simulink model "sampleModel2002_1_sub_sub"  (R2023a)
settings: Solver=VariableStepAuto  StartTime=0.0  StopTime=10.0  RelTol=1e-3
libraries: hdlsllib x9
settings Model: Creator=user1  LastModifiedBy=user1

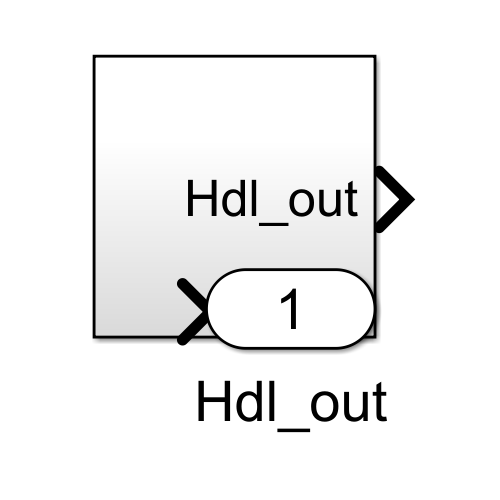
[thumbnail: Simulink's stored preview of the top-level diagram]
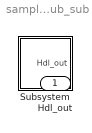
== system sampleModel2002_1_sub_sub ==
  Subsystem : Subsystem
  Hdl_out : Outport  OutDataTypeStr=uint8

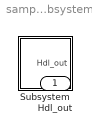
== system sampleModel2002_1_sub_sub/Subsystem ==
  Subsystem : Subsystem
  Hdl_out : Outport  OutDataTypeStr=uint8

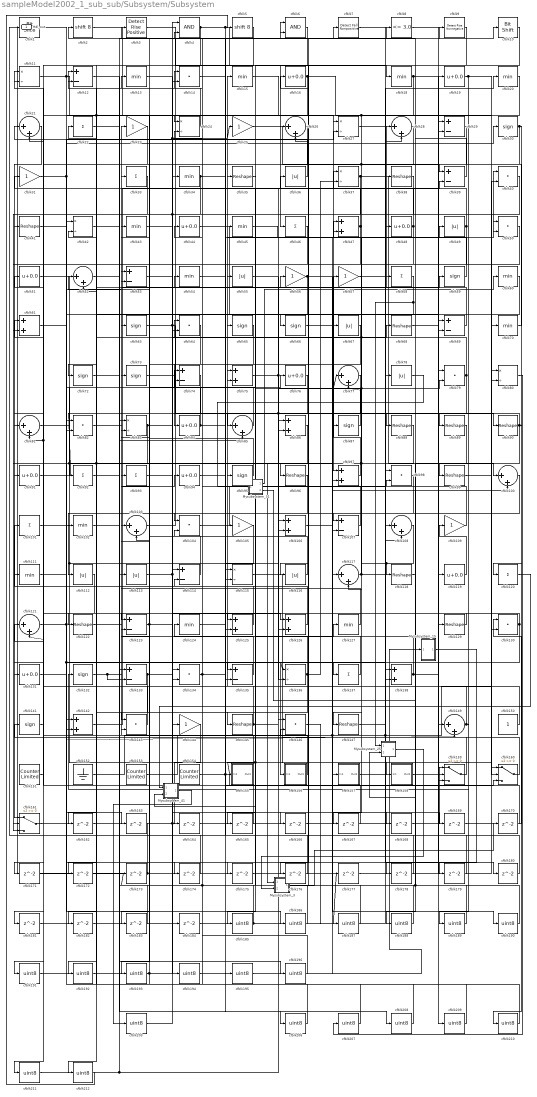
== system sampleModel2002_1_sub_sub/Subsystem/Subsystem ==
  Mysubsystem_15 : Subsystem  TreatAsAtomicUnit=on  RTWFcnName=Mysubsystem_15
      settings: RTWFcnNameOpts=User specified  RTWFileNameOpts=Use function name
  Mysubsystem_25 : Subsystem  TreatAsAtomicUnit=on  RTWFcnName=Mysubsystem_25
      settings: RTWFcnNameOpts=User specified  RTWFileNameOpts=Use function name
  Mysubsystem_3 : Subsystem  TreatAsAtomicUnit=on  RTWFcnName=Mysubsystem_3
      settings: RTWFcnNameOpts=User specified  RTWFileNameOpts=Use function name
  Mysubsystem_31 : Subsystem  TreatAsAtomicUnit=on  RTWFcnName=Mysubsystem_31
      settings: RTWFcnNameOpts=User specified  RTWFileNameOpts=Use function name
  Mysubsystem_41 : Subsystem  TreatAsAtomicUnit=on  RTWFcnName=Mysubsystem_41
      settings: RTWFcnNameOpts=User specified  RTWFileNameOpts=Use function name
  cfblk1 : hdlsllib/Logic and Bit Operations/Bit Slice  lidx=7  ridx=0
  cfblk10 : hdlsllib/Logic and Bit Operations/Bit Shift  mode=Shift Left Logical  N=0
  cfblk{21,26,28,52,77,81,85,100,103,108,117,121,149} (13 alike) : Sum  Inputs=|++  OutDataTypeStr=uint8
  cfblk{22,33,46,58,92..93,101,120,137} (9 alike) : Sum  Inputs=+  OutDataTypeStr=uint8
  cfblk{13,15,18,20,34,43,45,54,60,70,102,111,124,127} (14 alike) : MinMax  OutDataTypeStr=uint8
  cfblk{14,40,50,64,79,82,98,104,130,134,143,146} (12 alike) : DotProduct  OutDataTypeStr=uint8
  cfblk{23,25,31,56..57,105,109,144} (8 alike) : Gain  OutDataTypeStr=uint8
  cfblk{47,61,75,86,97,106,125..126,138,142} (10 alike) : Sum  OutDataTypeStr=uint8
  cfblk{12,29,39,53,69,74,107,114,123,133,135} (11 alike) : Sum  Inputs=+-  OutDataTypeStr=uint8
  cfblk{11,24,27,37,42,80,83,115,136} (9 alike) : Product  Inputs=*/  OutDataTypeStr=uint8  RndMeth=Zero  SaturateOnIntegerOverflow=on
  cfblk{36,49,55,67,78,112..113,116} (8 alike) : Abs  OutDataTypeStr=uint8  SaturateOnIntegerOverflow=off
  cfblk{35,38,41,68,88..90,96,99,118,122,129,145,147} (14 alike) : Reshape
  cfblk{16,19,44,48,51,76,84,91,94,119,131} (11 alike) : Bias  Bias=0.0  SaturateOnIntegerOverflow=off
  cfblk{30,59,63,65..66,72..73,87,95,132,141} (11 alike) : Signum
  cfblk150 : Constant  OutDataTypeStr=uint8  SampleTime=-1
  cfblk151 : hdlsllib/Sources/Counter Limited  uplimit=7  tsamp=-1
  cfblk152 : Ground
  cfblk153 : hdlsllib/Sources/Counter Limited  uplimit=7  tsamp=-1
  cfblk154 : hdlsllib/Sources/Counter Limited  uplimit=7  tsamp=-1
  cfblk155 : Subsystem
      settings: LibrarySourceBlock=|
      | hdlsllib/Ports &
      | Subsystems/Subsystem
  cfblk156 : Subsystem
      settings: LibrarySourceBlock=|
      | hdlsllib/Ports &
      | Subsystems/Subsystem
  cfblk157 : Subsystem
      settings: LibrarySourceBlock=|
      | hdlsllib/Ports &
      | Subsystems/Subsystem
  cfblk158 : Subsystem
      settings: LibrarySourceBlock=|
      | hdlsllib/Ports &
      | Subsystems/Subsystem
  cfblk159 : Switch  OutDataTypeStr=uint8  SaturateOnIntegerOverflow=off  InputSameDT=off
  cfblk160 : Switch  OutDataTypeStr=uint8  SaturateOnIntegerOverflow=off  InputSameDT=off
  cfblk161 : Switch  OutDataTypeStr=uint8  SaturateOnIntegerOverflow=off  InputSameDT=off
  cfblk{162..184} (23 alike) : Delay  SampleTime=1
  cfblk{185..196,203,206..212} (20 alike) : DataTypeConversion  OutDataTypeStr=uint8  SaturateOnIntegerOverflow=off  RndMeth=Floor
  cfblk2 : ArithShift  BitShiftNumber=8
  cfblk3 : hdlsllib/Logic and Bit Operations/Detect Rise Positive  vinit=0  OutDataTypeStr=uint8
  cfblk4 : Logic  AllPortsSameDT=off  OutDataTypeStr=boolean
  cfblk5 : ArithShift  BitShiftNumber=8
  cfblk6 : Logic  AllPortsSameDT=off  OutDataTypeStr=boolean
  cfblk7 : hdlsllib/Logic and Bit Operations/Detect Fall Nonpositive  vinit=0  OutDataTypeStr=uint8
  cfblk8 : hdlsllib/Logic and Bit Operations/Compare To Constant  relop=<=  const=3.0  OutDataTypeStr=uint8
  cfblk9 : hdlsllib/Logic and Bit Operations/Detect Rise Nonnegative  vinit=0  OutDataTypeStr=uint8
  Hdl_out : Outport  OutDataTypeStr=uint8
  wires:
  Mysubsystem_41/1(Out1) -> cfblk203/1
  cfblk120/1 -> Mysubsystem_41/1(In1)
  Mysubsystem_31/2(Out2) -> Mysubsystem_25/2(In2)
  Mysubsystem_31/1(Out1) -> cfblk60/1
  cfblk78/1 -> Mysubsystem_31/1(In1)
  Mysubsystem_25/1(Out1) -> Mysubsystem_3/2(In2)
  Mysubsystem_15/1(Out1) -> cfblk178/1
  cfblk195/1 -> Mysubsystem_15/1(In1)
  Mysubsystem_3/1(Out1) -> cfblk170/1
  cfblk212/1 -> cfblk5/1
  cfblk211/1 -> cfblk86/2, cfblk113/1
  cfblk210/1 -> cfblk42/2
  cfblk209/1 -> cfblk42/1
  cfblk8/1 -> cfblk209/1
  cfblk208/1 -> cfblk82/1
  cfblk42/1 -> cfblk208/1
  cfblk207/1 -> cfblk54/1
  cfblk80/1 -> cfblk207/1
  cfblk206/1 -> cfblk63/1
  cfblk54/1 -> cfblk206/1
  cfblk203/1 -> cfblk184/1
  cfblk196/1 -> cfblk124/1
  cfblk102/1 -> cfblk196/1
  cfblk124/1 -> cfblk195/1
  cfblk194/1 -> cfblk67/1
  cfblk43/1 -> cfblk194/1
  cfblk193/1 -> cfblk14/2, cfblk93/1
  cfblk192/1 -> cfblk106/2
  cfblk172/1 -> cfblk192/1
  cfblk191/1 -> cfblk106/1
  cfblk23/1 -> cfblk191/1
  cfblk190/1 -> cfblk98/2, cfblk43/1
  cfblk189/1 -> cfblk146/2
  cfblk188/1 -> cfblk146/1
  cfblk89/1 -> cfblk188/1
  cfblk187/1 -> cfblk173/1, cfblk104/2
  cfblk186/1 -> cfblk35/1
  cfblk61/1 -> cfblk186/1
  cfblk185/1 -> cfblk177/1, cfblk143/2
  cfblk184/1 -> cfblk117/1
  cfblk183/1 -> cfblk83/1
  cfblk182/1 -> cfblk133/1
  cfblk181/1 -> cfblk138/1
  cfblk26/1 -> cfblk181/1
  cfblk180/1 -> cfblk115/1
  cfblk27/1 -> cfblk180/1
  cfblk179/1 -> cfblk74/2
  cfblk178/1 -> cfblk123/2
  cfblk177/1 -> cfblk149/1
  cfblk176/1 -> cfblk24/2
  cfblk175/1 -> cfblk79/1
  cfblk52/1 -> cfblk175/1
  cfblk174/1 -> cfblk12/2
  cfblk173/1 -> cfblk142/1, Hdl_out/1
  cfblk171/1 -> cfblk130/2
  cfblk112/1 -> cfblk171/1
  cfblk170/1 -> cfblk103/1
  cfblk169/1 -> cfblk40/2
  cfblk157/1(Out1) -> cfblk169/1
  cfblk168/1 -> cfblk159/3
  cfblk14/1 -> cfblk168/1
  cfblk167/1 -> cfblk21/2
  cfblk166/1 -> cfblk29/2
  cfblk13/1 -> cfblk166/1
  cfblk165/1 -> cfblk121/1
  cfblk6/1 -> cfblk165/1
  cfblk164/1 -> cfblk108/2
  cfblk144/1 -> cfblk164/1
  cfblk163/1 -> cfblk1/1
  cfblk162/1 -> cfblk69/1
  cfblk46/1 -> cfblk61/2
  cfblk96/1 -> Mysubsystem_41/2(In2), cfblk155/1(In1)
  cfblk151/1 -> cfblk61/1
  cfblk90/1 -> cfblk87/1, cfblk99/1, cfblk120/1
  cfblk31/1 -> cfblk30/1, cfblk174/1
  cfblk50/1 -> cfblk135/2
  cfblk92/1 -> cfblk9/1
  cfblk147/1 -> cfblk20/1
  cfblk11/1 -> cfblk105/1, cfblk26/1
  cfblk7/1 -> cfblk98/1
  cfblk94/1 -> cfblk6/1
  cfblk66/1 -> cfblk50/1
  cfblk40/1 -> cfblk41/1
  cfblk58/1 -> Mysubsystem_25/1(In1), cfblk96/1
  cfblk60/1 -> cfblk117/2
  cfblk38/1 -> cfblk134/2, cfblk82/2
  cfblk20/1 -> cfblk103/2, cfblk77/2
  cfblk131/1 -> cfblk53/2
  cfblk22/1 -> cfblk138/2
  cfblk150/1 -> cfblk64/1
  cfblk123/1 -> cfblk126/1, cfblk83/2
  cfblk41/1 -> cfblk149/2, cfblk136/1
  cfblk99/1 -> cfblk80/2
  cfblk28/1 -> cfblk81/1, cfblk167/1
  cfblk24/1 -> cfblk12/1
  cfblk47/1 -> cfblk4/2, cfblk176/1
  cfblk117/1 -> cfblk77/1, cfblk47/2, cfblk48/1
  cfblk104/1 -> cfblk28/2
  cfblk83/1 -> cfblk59/1, cfblk131/1
  cfblk87/1 -> cfblk55/1
  cfblk12/1 -> cfblk85/2
  cfblk108/1 -> cfblk147/1, cfblk118/1
  cfblk49/1 -> cfblk116/1, cfblk11/2
  cfblk133/1 -> cfblk25/1, cfblk7/1, cfblk212/1
  cfblk160/1 -> cfblk141/1
  cfblk156/1(Out1) -> cfblk111/1
  cfblk111/1 -> cfblk27/2
  cfblk105/1 -> cfblk125/2
  cfblk69/1 -> cfblk22/1
  cfblk74/1 -> cfblk123/1
  cfblk55/1 -> cfblk86/1
  cfblk125/1 -> cfblk101/1
  cfblk15/1 -> cfblk27/1
  cfblk34/1 -> cfblk72/1, cfblk137/1
  cfblk19/1 -> cfblk160/1, cfblk189/1
  cfblk134/1 -> cfblk114/2, cfblk37/1
  cfblk95/1 -> cfblk53/1
  cfblk135/1 -> cfblk44/1
  cfblk143/1 -> cfblk31/1
  cfblk59/1 -> cfblk45/1
  cfblk116/1 -> cfblk52/1
  cfblk85/1 -> cfblk3/1
  cfblk65/1 -> cfblk143/1
  cfblk75/1 -> cfblk39/2, cfblk79/2
  cfblk142/1 -> cfblk127/1
  cfblk113/1 -> cfblk134/1, cfblk68/1
  cfblk35/1 -> cfblk185/1
  cfblk29/1 -> cfblk115/2
  cfblk64/1 -> cfblk84/1
  cfblk130/1 -> cfblk122/1, cfblk142/2
  cfblk33/1 -> cfblk161/3
  cfblk136/1 -> cfblk75/2, cfblk37/2, cfblk183/1
  cfblk100/1 -> cfblk112/1
  cfblk101/1 -> cfblk156/1(In1), cfblk126/2
  cfblk73/1 -> cfblk90/1
  cfblk3/1 -> cfblk108/1
  cfblk137/1 -> cfblk75/1
  cfblk67/1 -> cfblk193/1
  cfblk146/1 -> cfblk187/1
  cfblk98/1 -> cfblk104/1
  cfblk84/1 -> cfblk49/1, cfblk33/1
  cfblk129/1 -> cfblk125/1
  cfblk141/1 -> cfblk51/1
  cfblk5/1 -> cfblk211/1
  cfblk68/1 -> cfblk19/1
  cfblk56/1 -> cfblk100/2, cfblk172/1
  cfblk1/1 -> cfblk69/2
  cfblk10/1 -> cfblk18/1
  cfblk152/1 -> cfblk78/1, cfblk50/2, cfblk107/2
  cfblk18/1 -> cfblk121/2, cfblk81/2, cfblk162/1, cfblk160/2
  cfblk118/1 -> cfblk8/1
  cfblk30/1 -> cfblk89/1, cfblk210/1
  cfblk48/1 -> cfblk91/1, cfblk6/2
  cfblk36/1 -> cfblk13/1
  cfblk72/1 -> cfblk135/1
  cfblk138/1 -> cfblk29/1, cfblk26/2
  cfblk93/1 -> cfblk34/1
  cfblk161/1 -> cfblk130/1, cfblk4/1
  cfblk153/1 -> cfblk80/1
  cfblk126/1 -> cfblk95/1
  cfblk9/1 -> cfblk66/1
  cfblk76/1 -> cfblk145/1
  cfblk114/1 -> cfblk21/1
  cfblk79/1 -> cfblk52/2, cfblk47/1, cfblk88/1
  cfblk51/1 -> cfblk114/1
  cfblk109/1 -> cfblk14/1
  cfblk77/1 -> cfblk92/1, cfblk136/2
  cfblk86/1 -> cfblk161/2, cfblk182/1
  cfblk97/1 -> cfblk57/1
  cfblk37/1 -> cfblk100/1, cfblk64/2
  cfblk158/1(Out1) -> cfblk119/1
  cfblk16/1 -> cfblk24/1, cfblk70/1
  cfblk57/1 -> cfblk28/1
  cfblk159/1 -> cfblk16/1
  cfblk39/1 -> cfblk2/1
  cfblk25/1 -> cfblk129/1
  cfblk106/1 -> cfblk190/1
  cfblk149/1 -> cfblk132/1, cfblk11/1
  cfblk155/1(Out1) -> cfblk73/1
  cfblk91/1 -> cfblk76/1
  cfblk70/1 -> cfblk39/1
  cfblk115/1 -> cfblk159/2
  cfblk63/1 -> cfblk85/1, cfblk38/1
  cfblk53/1 -> cfblk144/1
  cfblk154/1 -> cfblk159/1, cfblk160/3
  cfblk81/1 -> cfblk158/1(In1), cfblk157/1(In1)
  cfblk122/1 -> cfblk36/1
  cfblk88/1 -> Mysubsystem_3/1(In1), cfblk107/1
  cfblk121/1 -> cfblk74/1, cfblk163/1
  cfblk44/1 -> cfblk97/2
  cfblk107/1 -> cfblk65/1
  cfblk82/1 -> cfblk56/1
  cfblk2/1 -> cfblk97/1
  cfblk21/1 -> cfblk161/1
  cfblk45/1 -> cfblk40/1
  cfblk132/1 -> cfblk94/1, cfblk133/2
  cfblk4/1 -> cfblk46/1, cfblk179/1, cfblk102/1
  cfblk145/1 -> cfblk15/1, cfblk58/1
  cfblk127/1 -> cfblk23/1
  cfblk119/1 -> cfblk109/1
  cfblk103/1 -> cfblk10/1

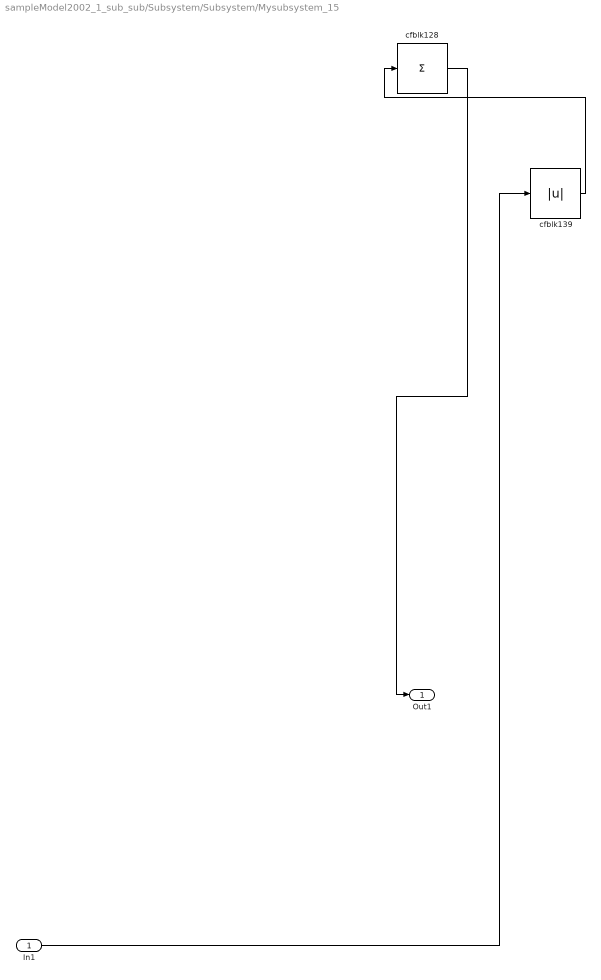
== system sampleModel2002_1_sub_sub/Subsystem/Subsystem/Mysubsystem_15 ==
  In1 : Inport
  cfblk128 : Sum  Inputs=+
  cfblk139 : Abs  SaturateOnIntegerOverflow=off
  Out1 : Outport
  wires:
  cfblk139/1 -> cfblk128/1
  In1/1 -> cfblk139/1
  cfblk128/1 -> Out1/1

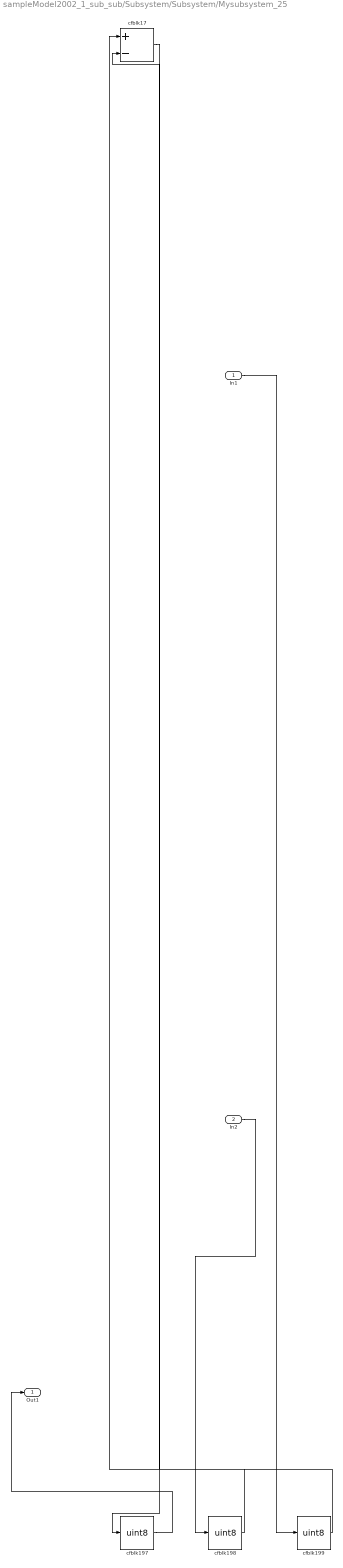
== system sampleModel2002_1_sub_sub/Subsystem/Subsystem/Mysubsystem_25 ==
  In1 : Inport
  In2 : Inport  Port=2
  cfblk17 : Sum  Inputs=+-
  cfblk197 : DataTypeConversion  OutDataTypeStr=uint8  SaturateOnIntegerOverflow=off  RndMeth=Floor
  cfblk198 : DataTypeConversion  OutDataTypeStr=uint8  SaturateOnIntegerOverflow=off  RndMeth=Floor
  cfblk199 : DataTypeConversion  OutDataTypeStr=uint8  SaturateOnIntegerOverflow=off  RndMeth=Floor
  Out1 : Outport
  wires:
  cfblk17/1 -> cfblk197/1
  In2/1 -> cfblk198/1
  cfblk198/1 -> cfblk17/1
  cfblk199/1 -> cfblk17/2
  In1/1 -> cfblk199/1
  cfblk197/1 -> Out1/1

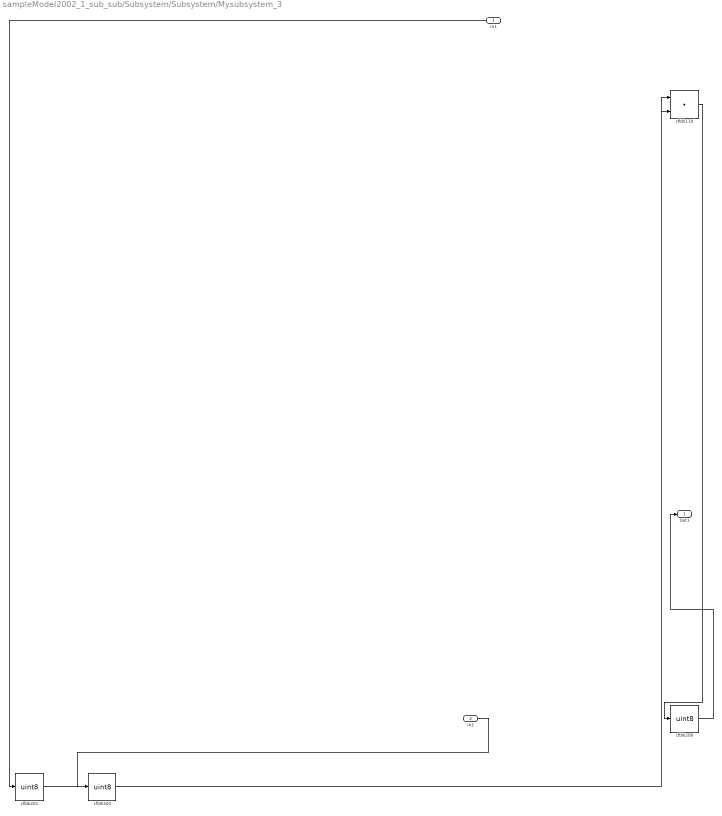
== system sampleModel2002_1_sub_sub/Subsystem/Subsystem/Mysubsystem_3 ==
  In1 : Inport
  In2 : Inport  Port=2
  cfblk110 : DotProduct  OutDataTypeStr=Inherit: Inherit via internal rule
  cfblk200 : DataTypeConversion  OutDataTypeStr=uint8  SaturateOnIntegerOverflow=off  RndMeth=Floor
  cfblk201 : DataTypeConversion  OutDataTypeStr=uint8  SaturateOnIntegerOverflow=off  RndMeth=Floor
  cfblk202 : DataTypeConversion  OutDataTypeStr=uint8  SaturateOnIntegerOverflow=off  RndMeth=Floor
  Out1 : Outport
  wires:
  In1/1 -> cfblk201/1
  cfblk202/1 -> cfblk110/2
  cfblk200/1 -> Out1/1
  In2/1 -> cfblk202/1
  cfblk110/1 -> cfblk200/1
  cfblk201/1 -> cfblk110/1

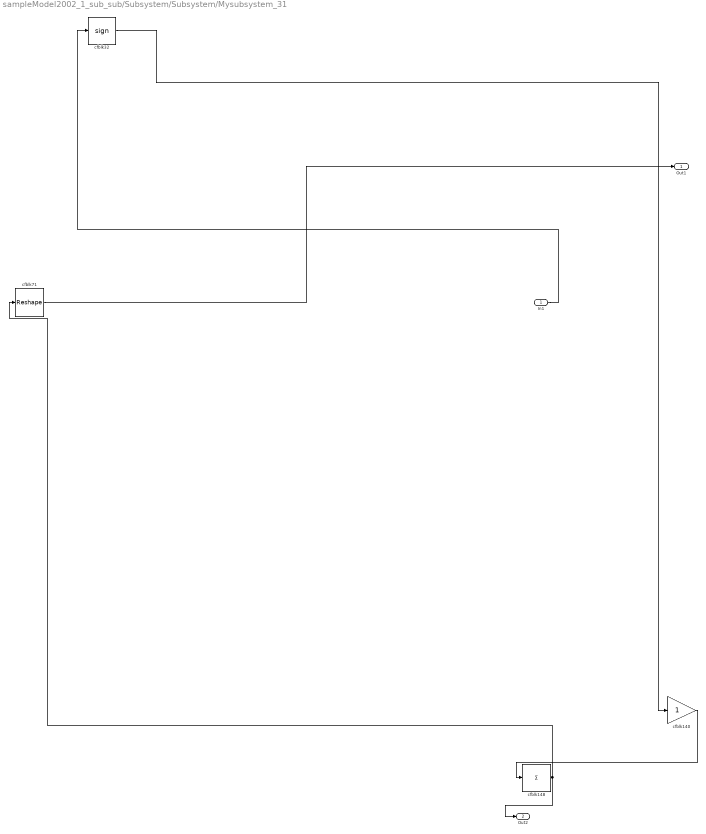
== system sampleModel2002_1_sub_sub/Subsystem/Subsystem/Mysubsystem_31 ==
  In1 : Inport
  cfblk140 : Gain
  cfblk148 : Sum  Inputs=+
  cfblk32 : Signum
  cfblk71 : Reshape
  Out1 : Outport
  Out2 : Outport  Port=2
  wires:
  cfblk148/1 -> Out2/1, cfblk71/1
  cfblk140/1 -> cfblk148/1
  cfblk32/1 -> cfblk140/1
  In1/1 -> cfblk32/1
  cfblk71/1 -> Out1/1

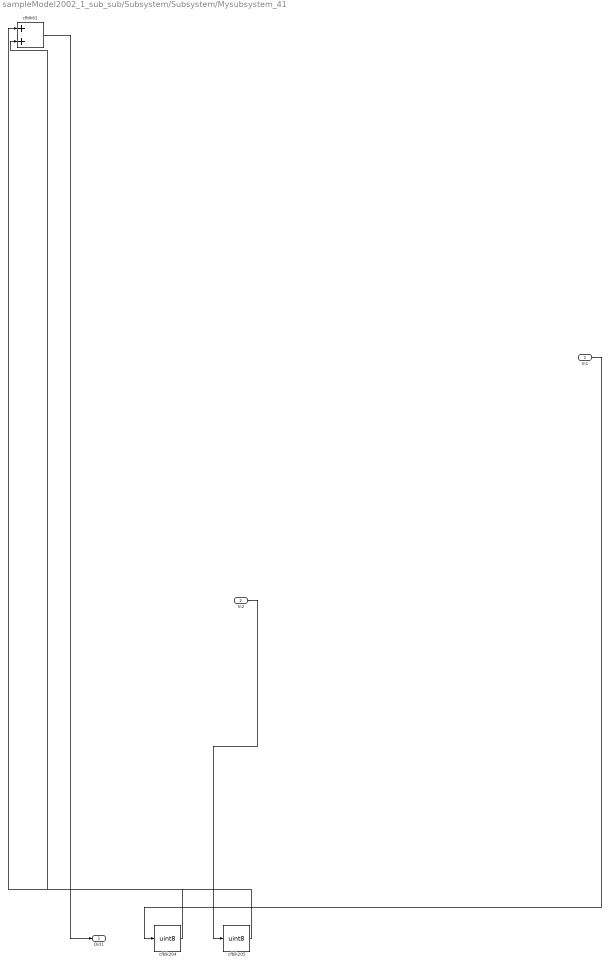
== system sampleModel2002_1_sub_sub/Subsystem/Subsystem/Mysubsystem_41 ==
  In1 : Inport
  In2 : Inport  Port=2
  cfblk204 : DataTypeConversion  OutDataTypeStr=uint8  SaturateOnIntegerOverflow=off  RndMeth=Floor
  cfblk205 : DataTypeConversion  OutDataTypeStr=uint8  SaturateOnIntegerOverflow=off  RndMeth=Floor
  cfblk62 : Sum
  Out1 : Outport
  wires:
  cfblk204/1 -> cfblk62/1
  cfblk205/1 -> cfblk62/2
  In2/1 -> cfblk205/1
  cfblk62/1 -> Out1/1
  In1/1 -> cfblk204/1

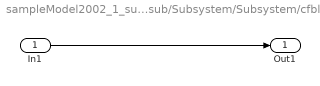
== system sampleModel2002_1_sub_sub/Subsystem/Subsystem/cfblk155 ==
  In1 : Inport
  Out1 : Outport
  wires:
  In1/1 -> Out1/1

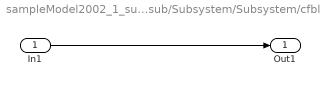
== system sampleModel2002_1_sub_sub/Subsystem/Subsystem/cfblk156 ==
  In1 : Inport
  Out1 : Outport
  wires:
  In1/1 -> Out1/1

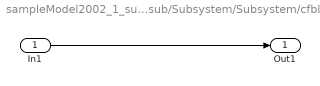
== system sampleModel2002_1_sub_sub/Subsystem/Subsystem/cfblk157 ==
  In1 : Inport
  Out1 : Outport
  wires:
  In1/1 -> Out1/1

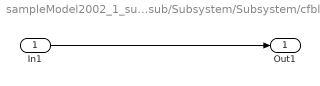
== system sampleModel2002_1_sub_sub/Subsystem/Subsystem/cfblk158 ==
  In1 : Inport
  Out1 : Outport
  wires:
  In1/1 -> Out1/1
